simulink model "controllo_v1"  (R2025b)
settings: Solver=VariableStepAuto  StartTime=0.0  StopTime=5  RelTol=1e-3
values from neighbouring files (symbols this model uses):
  a1 = 1.0    (= 1)    [init_robot.m]
  a2 = 1.0    (= 1)    [init_robot.m]
  a3 = 0.5    [init_robot.m]
  Fv = diag([0.1, 0.1, 0.1])    [init_robot.m]    (also in matrici_modello.m = diag([fv1, fv2, fv3]))
  g = 9.81    [init_robot.m]
  Il1 = (1/12)*ml1*a1^2    (= 0.416666666667)    [init_robot.m]
  Il2 = (1/12)*ml2*a2^2    (= 0.25)    [init_robot.m]
  Il3 = (1/12)*ml3*a3^2    (= 0.0208333333333)    [init_robot.m]
  Im1 = 0.01    [init_robot.m]
  Im2 = 0.01    [init_robot.m]
  Im3 = 0.01    [init_robot.m]
  Ki = diag([Ki_val, Ki_val, Ki_val])    [init_robot.m]
  Kp = diag([Kp_val, Kp_val, Kp_val])    [init_robot.m]
  kr1 = 50    [init_robot.m]
  kr2 = 50    [init_robot.m]
  kr3 = 50    [init_robot.m]
  Kv = diag([Kv_val, Kv_val, Kv_val])    [init_robot.m]
  l1 = a1/2    (= 0.5)    [init_robot.m]
  l2 = a2/2    (= 0.5)    [init_robot.m]
  l3 = a3/2    (= 0.25)    [init_robot.m]
  ml1 = 5.0    (= 5)    [init_robot.m]
  ml2 = 3.0    (= 3)    [init_robot.m]
  ml3 = 1.0    (= 1)    [init_robot.m]
  mm1 = 2.0    (= 2)    [init_robot.m]
  mm2 = 1.5    [init_robot.m]
  mm3 = 1.0    (= 1)    [init_robot.m]
settings Model: Creator=Utente  LastModifiedBy=W

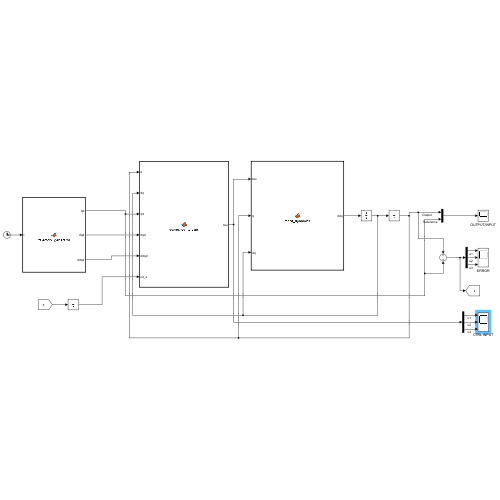
[thumbnail: Simulink's stored preview of the top-level diagram]
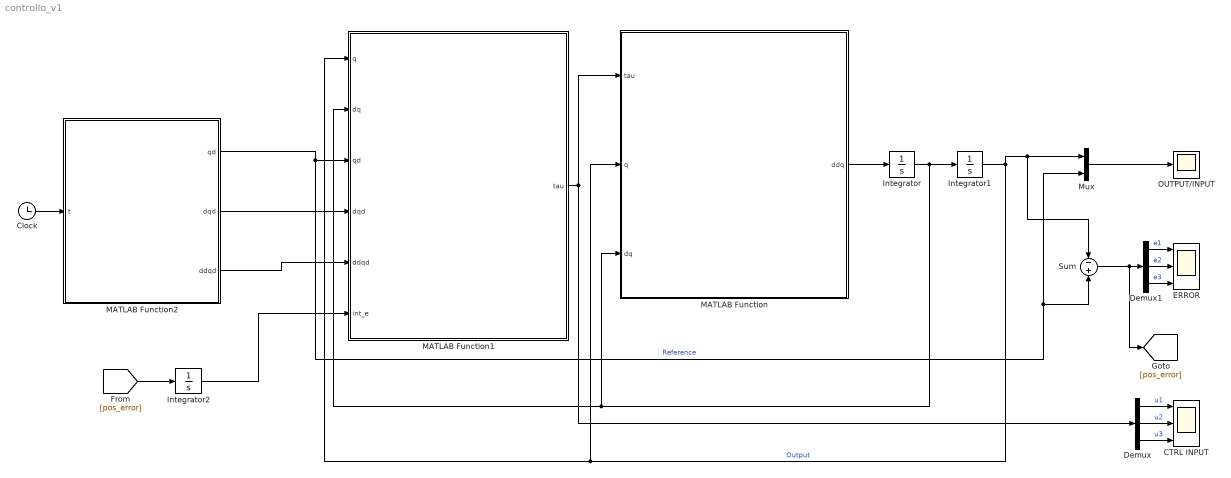
== system controllo_v1 ==
  CTRL INPUT : Scope  NumInputPorts=3
      settings: ActiveDisplayYMinimum=-226.46537402342966  ActiveDisplayYMaximum=436.54880697084815
  Clock : Clock
  Demux : Demux  Outputs=3
  Demux1 : Demux  Outputs=3
  ERROR : Scope  NumInputPorts=3
      settings: ActiveDisplayYMinimum=-0.003286558358802232  ActiveDisplayYMaximum=0.027131862726879757  DataLoggingVariableName=ScopeData2
  Integrator : Integrator
  Integrator1 : Integrator
  Integrator2 : Integrator
  MATLAB Function : MATLAB Function  TreatAsAtomicUnit=on
  MATLAB Function1 : MATLAB Function  TreatAsAtomicUnit=on
  MATLAB Function2 : MATLAB Function  TreatAsAtomicUnit=on
  Mux : Mux  Inputs=2
  OUTPUT/INPUT : Scope
      settings: ActiveDisplayYMinimum=-0.098816409308355835  ActiveDisplayYMaximum=0.883916133976131
  Sum : Sum  Inputs=-|+
  wires:
  MATLAB Function/1(ddq) -> Integrator/1
  MATLAB Function2/1(qd) -> Sum/2, Mux/2, MATLAB Function1/3(qd)  "Reference"
  MATLAB Function2/2(dqd) -> MATLAB Function1/4(dqd)
  MATLAB Function2/3(ddqd) -> MATLAB Function1/5(ddqd)
  Clock/1 -> MATLAB Function2/1(t)
  MATLAB Function1/1(tau) -> MATLAB Function/1(tau), Demux/1
  Demux/1 -> CTRL INPUT/1  "u1"
  Demux/2 -> CTRL INPUT/2  "u2"
  Demux/3 -> CTRL INPUT/3  "u3"
  Demux1/1 -> ERROR/1  "e1"
  Demux1/2 -> ERROR/2  "e2"
  Demux1/3 -> ERROR/3  "e3"
  Sum/1 -> [pos_error], Demux1/1
  Mux/1 -> OUTPUT/INPUT/1
  Integrator/1 -> Integrator1/1, MATLAB Function1/2(dq), MATLAB Function/3(dq)
  Integrator1/1 -> Mux/1, Sum/1, MATLAB Function1/1(q), MATLAB Function/2(q)  "Output"
  [pos_error] -> Integrator2/1
  Integrator2/1 -> MATLAB Function1/6(int_e)

== matlab function controllo_v1/MATLAB Function ==
  data: tau input; ddq output; q input; dq input; a1 parameter; a2 parameter; a3 parameter; l1 parameter; l2 parameter; l3 parameter; ml1 parameter; ml2 parameter; ml3 parameter; mm1 parameter; mm2 parameter; mm3 parameter; Il1 parameter; Il2 parameter; Il3 parameter; Im1 parameter; Im2 parameter; Im3 parameter; kr1 parameter; kr2 parameter; kr3 parameter; g parameter; Fv parameter
function ddq = robot_dynamics(tau, q, dq, a1, a2, a3, l1, l2, l3, ml1, ml2, ml3, mm1, mm2, mm3, Il1, Il2, Il3, Im1, Im2, Im3, kr1, kr2, kr3, g, Fv)
    % --- PRE-ALLOCATION ---
    ddq = zeros(3,1);        
    
    % Call the exported dynamic matrices (Physical Plant model)
    B = calc_B(q, a1, a2, a3, l1, l2, l3, ml1, ml2, ml3, mm1, mm2, mm3, Il1, Il2, Il3, Im1, Im2, Im3, kr1, kr2, kr3);
    C = calc_C(q, dq, a1, a2, a3, l1, l2, l3, ml1, ml2, ml3, mm1, mm2, mm3, Il1, Il2, Il3, Im1, Im2, Im3, kr1, kr2, kr3);
    G_v = calc_G(q, g, a1, a2, a3, l1, l2, l3, ml1, ml2, ml3, mm1, mm2, mm3);
    
    % Solve the forward dynamics equation to find the joint accelerations
    % Equation: B*ddq + C*dq + G + Fv*dq = tau 
    % Solution: ddq = B \ (tau - C*dq - G_v - Fv*dq)
    
    ddq = B \ (tau - C*dq - G_v - Fv*dq); % Compute ddq: we consider Fs = 0 and no external forces
end

== matlab function controllo_v1/MATLAB Function2 ==
  data: t input; qd output; dqd output; ddqd output
function [qd, dqd, ddqd] = trajectory_generator(t)
    % Initialize output vectors
    qd = zeros(3,1);    
    dqd = zeros(3,1);    
    ddqd = zeros(3,1);    
    
    % -----------------------------------------------------------------
    % OPTION 1: Simple Synchronous Oscillation (45 degrees)
    % -----------------------------------------------------------------
    % A = pi/4; % Amplitude (45 degrees)
    % w = 1.0;  % Pulsation (rad/s)
    % 
    % qd = [A * sin(w*t); 
    %       A * sin(w*t); 
    %       A * sin(w*t)];
    % 
    % dqd = [A * w * cos(w*t); 
    %        A * w * cos(w*t); 
    %        A * w * cos(w*t)];
    % 
    % ddqd = [-A * w^2 * sin(w*t); 
    %         -A * w^2 * sin(w*t); 
    %         -A * w^2 * sin(w*t)];
    
    % -----------------------------------------------------------------
    % OPTION 2: Independent Oscillations for each joint
    % -----------------------------------------------------------------
    % A1 = pi/4;  w1 = 1.0;   % Joint 1
    % A2 = pi/6;  w2 = 2.0;   % Joint 2
    % A3 = pi/8;  w3 = 0.5;   % Joint 3
    % 
    % qd = [A1 * sin(w1*t); 
    %       A2 * sin(w2*t); 
    %       A3 * sin(w3*t)];
    % 
    % dqd = [A1 * w1 * cos(w1*t); 
    %        A2 * w2 * cos(w2*t); 
    %        A3 * w3 * cos(w3*t)];
    % 
    % ddqd = [-A1 * w1^2 * sin(w1*t); 
    %         -A2 * w2^2 * sin(w2*t); 
    %         -A3 * w3^2 * sin(w3*t)];  
    
    % -----------------------------------------------------------------
    % OPTION 3: Constant Step Reference (45 degrees)
    % Used for transient response analysis and gain tuning
    % -----------------------------------------------------------------
    % A = pi/4; 
    % qd = [A; 2*A; A];
    % dqd = [0; 0; 0];
    % ddqd = [0; 0; 0];
    
    % -----------------------------------------------------------------
    % OPTION 4: Quintic Polynomial Trajectory (Point-to-Point)
    % Smooth movement followed by a steady-state phase
    % -----------------------------------------------------------------
    tf = 1; % Final time for the quintic rise phase
    q_start = [0; 0; 0];
    q_end = [pi/4; pi/4; pi/4]; % Target: 45 degrees for all joints

    if t <= tf
        % Normalized time (tau = t/tf) for polynomial calculation
        tau = t/tf;
        A_diff = q_end - q_start;

        % 5th degree polynomial coefficients
        poly   = 10*tau^3 - 15*tau^4 + 6*tau^5;
        dpoly  = (30*tau^2 - 60*tau^3 + 30*tau^4) / tf;
        ddpoly = (60*tau - 180*tau^2 + 120*tau^3) / tf^2;

        qd   = q_start + A_diff * poly;
        dqd  = A_diff * dpoly;
        ddqd = A_diff * ddpoly;
    else
        % Steady-state phase: maintain target position
        qd   = q_end;
        dqd  = [0; 0; 0];
        ddqd = [0; 0; 0];
    end    
    
end

== matlab function controllo_v1/MATLAB Function1 ==
  data: q input; dq input; qd input; dqd input; ddqd input; int_e input; Kp parameter; Kv parameter; Ki parameter; a1 parameter; a2 parameter; a3 parameter; l1 parameter; l2 parameter; ml1 parameter; l3 parameter; ml2 parameter; ml3 parameter; mm1 parameter; mm2 parameter; mm3 parameter; Il1 parameter; Il2 parameter; Il3 parameter; Im1 parameter; Im2 parameter; Im3 parameter; kr1 parameter; kr2 parameter; kr3 parameter; g parameter; Fv parameter; tau output size=[3, 1]
function tau = computed_torque(q, dq, qd, dqd, ddqd, int_e, Kp, Kv, Ki, a1, a2, a3, l1, l2, ml1, l3, ml2, ml3, mm1, mm2, mm3, Il1, Il2, Il3, Im1, Im2, Im3, kr1, kr2, kr3, g, Fv)
    % --- PRE-ALLOCATION FOR SIMULINK ---
    tau = zeros(3,1);
    % Ki = 0;
    % Internal Model parameters (Estimated masses used by the controller)
    % Note: These can differ from the actual plant masses (ml1, ml2, ml3) to test robustness
    ml1_est = 0.2 * ml1; 
    ml2_est = 0.2 * ml2; 
    ml3_est = 0.2 * ml3;

    
    % Recalculate B, C, and G matrices based on the estimated internal model
    B = calc_B(q, a1, a2, a3, l1, l2, l3, ml1_est, ml2_est, ml3_est, mm1, mm2, mm3, Il1, Il2, Il3, Im1, Im2, Im3, kr1, kr2, kr3);
    C = calc_C(q, dq, a1, a2, a3, l1, l2, l3, ml1_est, ml2_est, ml3_est, mm1, mm2, mm3, Il1, Il2, Il3, Im1, Im2, Im3, kr1, kr2, kr3);
    G_v = calc_G(q, g, a1, a2, a3, l1, l2, l3, ml1_est, ml2_est, ml3_est, mm1, mm2, mm3);
    
    % Calculate tracking errors (Position, Velocity, and Integral)
    e = qd - q;
    de = dqd - dq;
    
    % Linear Control Law (PID structure in the joint space)
    % According to the Robust Feedback Linearization approach (Lewis et al.)
    % v = ddqd + Kv*de + Kp*e + Ki*int_e
    v = ddqd + Kv*de + Kp*e + Ki*int_e;
    
    % Final Control Torque Computation
    % tau = B * v + C*dq + G + Fv*dq
    tau = B * v + C*dq + G_v + Fv*dq;
end
